simulink model "LimbIdentification"  (R2018b)
settings: Solver=FixedStepAuto  StartTime=0.0  StopTime=1250.0  FixedStep=Ts  RelTol=1e-3
InitFcn:
  | init
values from neighbouring files (symbols this model uses):
  m = 1    [gpcData.mat]
undefined symbols (not defined in the file or in its folder): B1, B2, B3, g, J, K1, K2, K3, l, Td
libraries: simulink x3
settings Model: Creator=hhhhh  LastModifiedBy=root

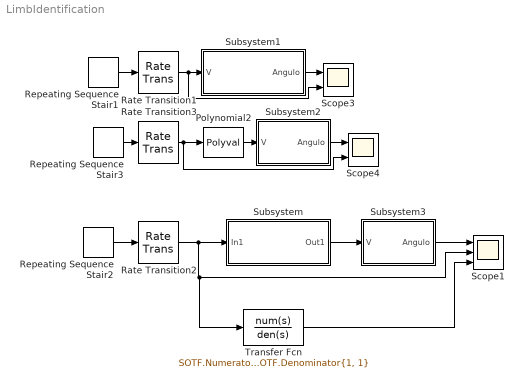
== system LimbIdentification ==
  Polynomial2 : Polyval  Coefs=|
      | [0.456167901712123
      | 0
      | 0
      | 0
      | 1.92078367330958
      | 0
      | 0
      | 4.34814267315048
      | 0
      | 11.9677550168665
      | 0]
  Rate Transition1 : RateTransition
  Rate Transition2 : RateTransition
  Rate Transition3 : RateTransition
  Repeating Sequence Stair1 : simulink/Sources/Repeating Sequence Stair  OutValues="50*[0\t0.0523359562429438\t0.104528463267653\t0.156434465040231\t0.207911690817759\t0.258819045102521\t0.309016994374947\t0.358367949545300\t0.406736643075800\t0.453990499739547\t0.500000000000000\t0.544639035015027\t0.587785252292473\t0.629320391049837\t0.669130606358858\t0.707106781186548\t0.743144825477394\t0.777145961456971\t0.809016994374948\t0.838670567945424\t0.866025403784439\t0.891006524188368\t0.913545457642601\t0.933580426497202\t0.951056516295154\t0.965925826289068\t0.978147600733806\t0.987688340595138\t0.994521895368273\t0.998629534754574\t1\t0.998629534754574\t0.994521895368273\t0.987688340595138\t0.978147600733806\t0.965925826289068\t0.951056516295154\t0.933580426497202\t0.913545457642601\t0.891006524188368\t0.866025403784439\t0.838670567945424\t0.809016994374948\t0.777145961456971\t0.743144825477394\t0.707106781186548\t0.669130606358858\t0.629320391049837\t0.587785252292473\t0.544639035015027\t0.500000000000000\t0.453990499739547\t0.406736643075800\t0.358367949545300\t0.309016994374948\t0.258819045102521\t0.207911690817759\t0.156434465040231\t0.104528463267654\t0.0523359562429438].'"  tsamp=20  OutMin=[]  OutMax=[]  OutDataTypeStr=double  OutputDataTypeScalingMode=double  OutDataType=fixdt(0,8)  ConRadixGroup=Best Precision: Vector-wise  OutScaling=2^-12
  Repeating Sequence Stair2 : simulink/Sources/Repeating Sequence Stair  OutValues="1.3*[0\t0.0523359562429438\t0.104528463267653\t0.156434465040231\t0.207911690817759\t0.258819045102521\t0.309016994374947\t0.358367949545300\t0.406736643075800\t0.453990499739547\t0.500000000000000\t0.544639035015027\t0.587785252292473\t0.629320391049837\t0.669130606358858\t0.707106781186548\t0.743144825477394\t0.777145961456971\t0.809016994374948\t0.838670567945424\t0.866025403784439\t0.891006524188368\t0.913545457642601\t0.933580426497202\t0.951056516295154\t0.965925826289068\t0.978147600733806\t0.987688340595138\t0.994521895368273\t0.998629534754574\t1\t0.998629534754574\t0.994521895368273\t0.987688340595138\t0.978147600733806\t0.965925826289068\t0.951056516295154\t0.933580426497202\t0.913545457642601\t0.891006524188368\t0.866025403784439\t0.838670567945424\t0.809016994374948\t0.777145961456971\t0.743144825477394\t0.707106781186548\t0.669130606358858\t0.629320391049837\t0.587785252292473\t0.544639035015027\t0.500000000000000\t0.453990499739547\t0.406736643075800\t0.358367949545300\t0.309016994374948\t0.258819045102521\t0.207911690817759\t0.156434465040231\t0.104528463267654\t0.0523359562429438].'"  tsamp=20  OutMin=[]  OutMax=[]  OutDataTypeStr=double  OutputDataTypeScalingMode=double  OutDataType=fixdt(0,8)  ConRadixGroup=Best Precision: Vector-wise  OutScaling=2^-12
  Repeating Sequence Stair3 : simulink/Sources/Repeating Sequence Stair  OutValues="0.5*[0\t0.0523359562429438\t0.104528463267653\t0.156434465040231\t0.207911690817759\t0.258819045102521\t0.309016994374947\t0.358367949545300\t0.406736643075800\t0.453990499739547\t0.500000000000000\t0.544639035015027\t0.587785252292473\t0.629320391049837\t0.669130606358858\t0.707106781186548\t0.743144825477394\t0.777145961456971\t0.809016994374948\t0.838670567945424\t0.866025403784439\t0.891006524188368\t0.913545457642601\t0.933580426497202\t0.951056516295154\t0.965925826289068\t0.978147600733806\t0.987688340595138\t0.994521895368273\t0.998629534754574\t1\t0.998629534754574\t0.994521895368273\t0.987688340595138\t0.978147600733806\t0.965925826289068\t0.951056516295154\t0.933580426497202\t0.913545457642601\t0.891006524188368\t0.866025403784439\t0.838670567945424\t0.809016994374948\t0.777145961456971\t0.743144825477394\t0.707106781186548\t0.669130606358858\t0.629320391049837\t0.587785252292473\t0.544639035015027\t0.500000000000000\t0.453990499739547\t0.406736643075800\t0.358367949545300\t0.309016994374948\t0.258819045102521\t0.207911690817759\t0.156434465040231\t0.104528463267654\t0.0523359562429438].'"  tsamp=20  OutMin=[]  OutMax=[]  OutDataTypeStr=double  OutputDataTypeScalingMode=double  OutDataType=fixdt(0,8)  ConRadixGroup=Best Precision: Vector-wise  OutScaling=2^-12
  Scope1 : Scope  NumInputPorts=3
  Scope3 : Scope  NumInputPorts=2
  Scope4 : Scope  NumInputPorts=2
  Subsystem : Subsystem
  Subsystem1 : Subsystem
  Subsystem2 : Subsystem
  Subsystem3 : Subsystem
  Transfer Fcn : TransferFcn  Numerator=SOTF.Numerator{1, 1}  Denominator=SOTF.Denominator{1, 1}
  wires:
  Subsystem1/1(Angulo) -> Scope3/1
  Rate Transition1/1 -> Scope3/2, Subsystem1/1(V)
  Polynomial2/1 -> Subsystem2/1(V)
  Subsystem2/1(Angulo) -> Scope4/1
  Repeating Sequence Stair1/1 -> Rate Transition1/1
  Repeating Sequence Stair3/1 -> Rate Transition3/1
  Rate Transition3/1 -> Polynomial2/1, Scope4/2
  Rate Transition2/1 -> Subsystem/1(In1), Transfer Fcn/1, Scope1/2
  Repeating Sequence Stair2/1 -> Rate Transition2/1
  Subsystem3/1(Angulo) -> Scope1/1
  Subsystem/1(Out1) -> Subsystem3/1(V)
  Transfer Fcn/1 -> Scope1/3

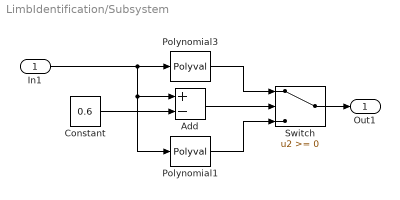
== system LimbIdentification/Subsystem ==
  In1 : Inport
  Add : Sum  Inputs=+-
  Constant : Constant  Value=0.6
  Polynomial1 : Polyval  Coefs=|
      | [0
      | 0
      | 0
      | 4.96473696106646
      | 0
      | 1.22506777764656
      | 11.8762695363768
      | 0]
  Polynomial3 : Polyval  Coefs=|
      | [1334.93659745298
      | -7873.77408130260
      | 19679.6581173489
      | -26904.1335294621
      | 21674.5719980287
      | -10255.6450049827
      | 2645.19572957251
      | -282.136494548769]
  Switch : Switch
  Out1 : Outport
  wires:
  Switch/1 -> Out1/1
  In1/1 -> Add/1, Polynomial1/1, Polynomial3/1
  Constant/1 -> Add/2
  Add/1 -> Switch/2
  Polynomial3/1 -> Switch/1
  Polynomial1/1 -> Switch/3

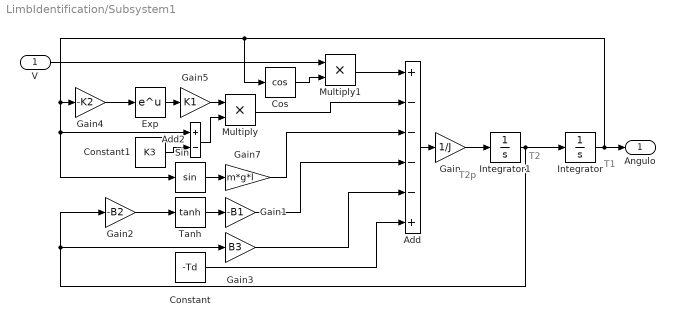
== system LimbIdentification/Subsystem1 ==
  note: T1
  note: T2p
  note: T2
  V : Inport
  Add : Sum  Inputs=+----+
  Add2 : Sum  Inputs=+-
  Constant : Constant  Value=-Td
  Constant1 : Constant  Value=K3
  Cos : Trigonometry  Operator=cos
  Exp : Math  SaturateOnIntegerOverflow=on
  Gain : Gain  Gain=1/J
  Gain1 : Gain  Gain=-B1
  Gain2 : Gain  Gain=-B2
  Gain3 : Gain  Gain=B3
  Gain4 : Gain  Gain=-K2
  Gain5 : Gain  Gain=K1
  Gain7 : Gain  Gain=m*g*l
  Integrator : Integrator
  Integrator1 : Integrator
  Multiply : Product
  Multiply1 : Product
  Sin : Trigonometry
  Tanh : Trigonometry  Operator=tanh
  Angulo : Outport
  wires:
  Integrator/1 -> Gain4/1, Add2/1, Sin/1, Cos/1, Angulo/1
  Gain2/1 -> Tanh/1
  Integrator1/1 -> Gain2/1, Gain3/1, Integrator/1
  Exp/1 -> Gain5/1
  Gain7/1 -> Add/3
  Sin/1 -> Gain7/1
  V/1 -> Multiply1/1
  Add2/1 -> Multiply/2
  Multiply1/1 -> Add/1
  Gain4/1 -> Exp/1
  Multiply/1 -> Add/2
  Tanh/1 -> Gain1/1
  Add/1 -> Gain/1
  Cos/1 -> Multiply1/2
  Gain3/1 -> Add/5
  Constant/1 -> Add/6
  Gain1/1 -> Add/4
  Gain5/1 -> Multiply/1
  Gain/1 -> Integrator1/1
  Constant1/1 -> Add2/2

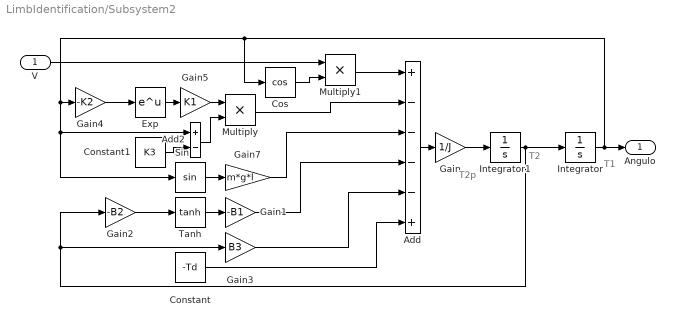
== system LimbIdentification/Subsystem2 ==
  note: T2
  note: T2p
  note: T1
  V : Inport
  Add : Sum  Inputs=+----+
  Add2 : Sum  Inputs=+-
  Constant : Constant  Value=-Td
  Constant1 : Constant  Value=K3
  Cos : Trigonometry  Operator=cos
  Exp : Math  SaturateOnIntegerOverflow=on
  Gain : Gain  Gain=1/J
  Gain1 : Gain  Gain=-B1
  Gain2 : Gain  Gain=-B2
  Gain3 : Gain  Gain=B3
  Gain4 : Gain  Gain=-K2
  Gain5 : Gain  Gain=K1
  Gain7 : Gain  Gain=m*g*l
  Integrator : Integrator
  Integrator1 : Integrator
  Multiply : Product
  Multiply1 : Product
  Sin : Trigonometry
  Tanh : Trigonometry  Operator=tanh
  Angulo : Outport
  wires:
  Constant1/1 -> Add2/2
  Gain/1 -> Integrator1/1
  Gain5/1 -> Multiply/1
  Gain1/1 -> Add/4
  Constant/1 -> Add/6
  Gain3/1 -> Add/5
  Cos/1 -> Multiply1/2
  Add/1 -> Gain/1
  Tanh/1 -> Gain1/1
  Multiply/1 -> Add/2
  Gain4/1 -> Exp/1
  Multiply1/1 -> Add/1
  Add2/1 -> Multiply/2
  V/1 -> Multiply1/1
  Sin/1 -> Gain7/1
  Gain7/1 -> Add/3
  Exp/1 -> Gain5/1
  Integrator1/1 -> Integrator/1, Gain3/1, Gain2/1
  Gain2/1 -> Tanh/1
  Integrator/1 -> Angulo/1, Cos/1, Sin/1, Add2/1, Gain4/1

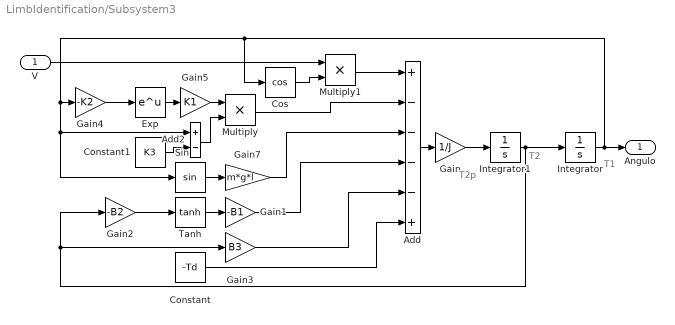
== system LimbIdentification/Subsystem3 ==
  note: T1
  note: T2p
  note: T2
  V : Inport
  Add : Sum  Inputs=+----+
  Add2 : Sum  Inputs=+-
  Constant : Constant  Value=-Td
  Constant1 : Constant  Value=K3
  Cos : Trigonometry  Operator=cos
  Exp : Math  SaturateOnIntegerOverflow=on
  Gain : Gain  Gain=1/J
  Gain1 : Gain  Gain=-B1
  Gain2 : Gain  Gain=-B2
  Gain3 : Gain  Gain=B3
  Gain4 : Gain  Gain=-K2
  Gain5 : Gain  Gain=K1
  Gain7 : Gain  Gain=m*g*l
  Integrator : Integrator
  Integrator1 : Integrator
  Multiply : Product
  Multiply1 : Product
  Sin : Trigonometry
  Tanh : Trigonometry  Operator=tanh
  Angulo : Outport
  wires:
  Integrator/1 -> Gain4/1, Add2/1, Sin/1, Cos/1, Angulo/1
  Gain2/1 -> Tanh/1
  Integrator1/1 -> Gain2/1, Gain3/1, Integrator/1
  Exp/1 -> Gain5/1
  Gain7/1 -> Add/3
  Sin/1 -> Gain7/1
  V/1 -> Multiply1/1
  Add2/1 -> Multiply/2
  Multiply1/1 -> Add/1
  Gain4/1 -> Exp/1
  Multiply/1 -> Add/2
  Tanh/1 -> Gain1/1
  Add/1 -> Gain/1
  Cos/1 -> Multiply1/2
  Gain3/1 -> Add/5
  Constant/1 -> Add/6
  Gain1/1 -> Add/4
  Gain5/1 -> Multiply/1
  Gain/1 -> Integrator1/1
  Constant1/1 -> Add2/2
